simulink model "incrimental_couter_using_basics_blocks"  (R2020a)
settings: Solver=VariableStepAuto  StartTime=0.0  StopTime=10.0  RelTol=1e-3
settings Model: Creator=Kundan Patil  LastModifiedBy=Kundan Patil

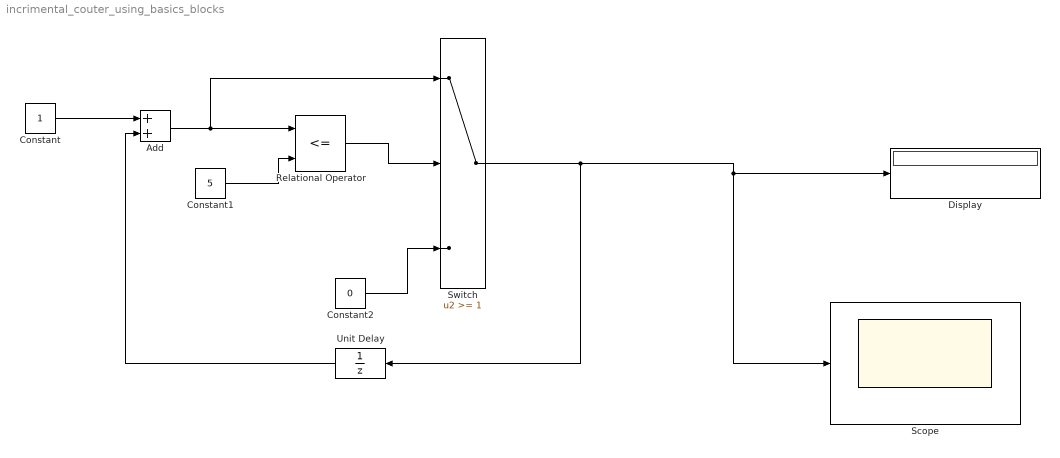
== system incrimental_couter_using_basics_blocks ==
  Add : Sum
  Constant : Constant
  Constant1 : Constant  Value=5
  Constant2 : Constant  Value=0
  Display : Display
  Relational Operator : RelationalOperator  Operator=<=  OutDataTypeStr=boolean  RndMeth=Simplest
  Scope : Scope
  Switch : Switch  Threshold=1
  Unit Delay : UnitDelay  InitialCondition=-1  SampleTime=-1  HasFrameUpgradeWarning=on
  wires:
  Relational Operator/1 -> Switch/2
  Switch/1 -> Scope/1, Display/1, Unit Delay/1
  Constant/1 -> Add/1
  Constant1/1 -> Relational Operator/2
  Unit Delay/1 -> Add/2
  Add/1 -> Relational Operator/1, Switch/1
  Constant2/1 -> Switch/3
